simulink model "digital9adder"  (R2024a)
settings: Solver=VariableStepAuto  StartTime=0.0  StopTime=10.0  RelTol=1e-3
settings Model: Creator=tusha  LastModifiedBy=tusha

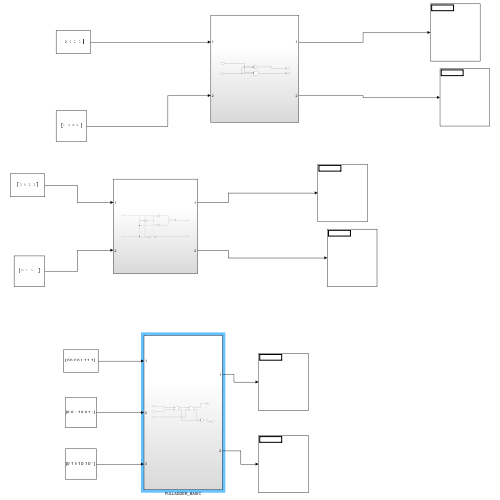
[thumbnail: Simulink's stored preview of the top-level diagram]
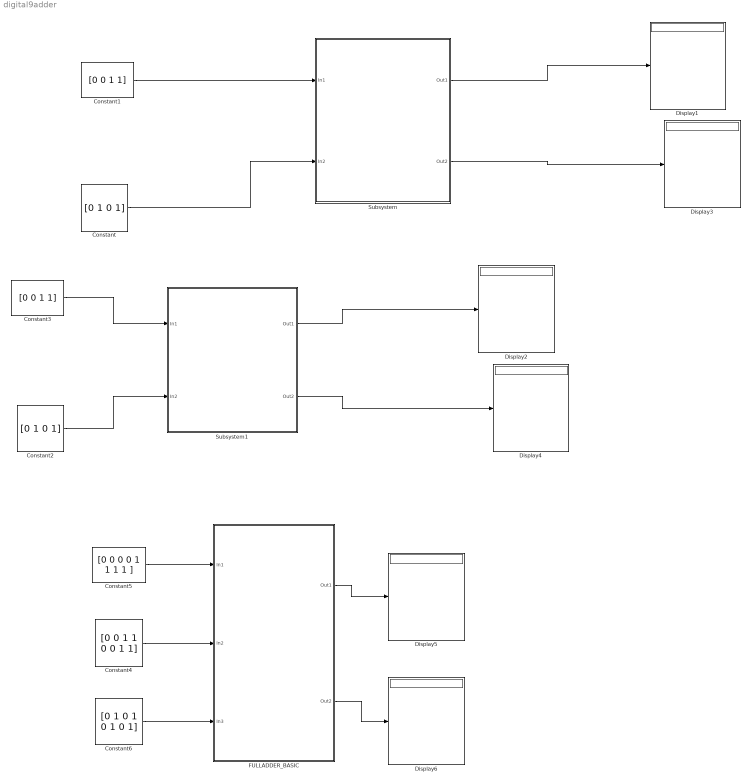
== system digital9adder ==
  Constant : Constant  Value=[0 1 0 1]
  Constant1 : Constant  Value=[0 0 1 1]
  Constant2 : Constant  Value=[0 1 0 1]
  Constant3 : Constant  Value=[0 0 1 1]
  Constant4 : Constant  Value=[0 0 1 1 0 0 1 1]
  Constant5 : Constant  Value=[0 0 0 0 1 1 1 1 ]
  Constant6 : Constant  Value=[0 1 0 1 0 1 0 1]
  Display{1..6} (6 alike) : Display
  FULLADDER_BASIC : Subsystem
  Subsystem : Subsystem
  Subsystem1 : Subsystem
  wires:
  Constant1/1 -> Subsystem/1(In1)
  Constant/1 -> Subsystem/2(In2)
  Subsystem/2(Out2) -> Display3/1
  Subsystem/1(Out1) -> Display1/1
  Constant3/1 -> Subsystem1/1(In1)
  Constant2/1 -> Subsystem1/2(In2)
  Subsystem1/1(Out1) -> Display2/1
  Subsystem1/2(Out2) -> Display4/1
  Constant5/1 -> FULLADDER_BASIC/1(In1)
  Constant4/1 -> FULLADDER_BASIC/2(In2)
  Constant6/1 -> FULLADDER_BASIC/3(In3)
  FULLADDER_BASIC/1(Out1) -> Display5/1
  FULLADDER_BASIC/2(Out2) -> Display6/1

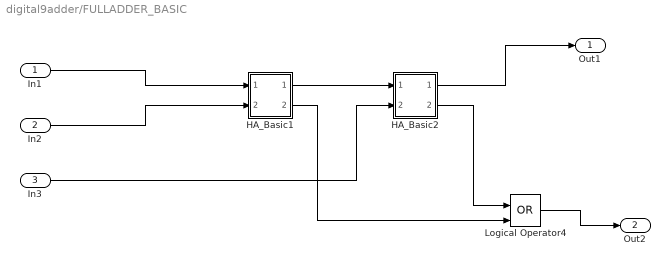
== system digital9adder/FULLADDER_BASIC ==
  In1 : Inport
  In2 : Inport  Port=2
  In3 : Inport  Port=3
  HA_Basic1 : Subsystem
  HA_Basic2 : Subsystem
  Logical Operator4 : Logic  Operator=OR  IconShape=distinctive  AllPortsSameDT=off  OutDataTypeStr=boolean
  Out1 : Outport
  Out2 : Outport  Port=2
  wires:
  HA_Basic1/1(Out1) -> HA_Basic2/1(In1)
  HA_Basic1/2(Out2) -> Logical Operator4/2
  HA_Basic2/2(Out2) -> Logical Operator4/1
  In1/1 -> HA_Basic1/1(In1)
  Logical Operator4/1 -> Out2/1
  In2/1 -> HA_Basic1/2(In2)
  HA_Basic2/1(Out1) -> Out1/1
  In3/1 -> HA_Basic2/2(In2)

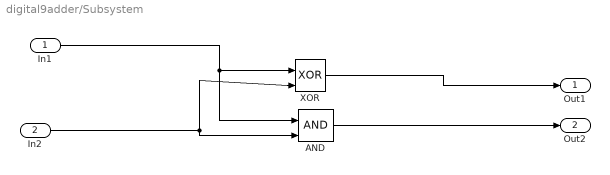
== system digital9adder/Subsystem ==
  In1 : Inport
  In2 : Inport  Port=2
  AND : Logic  IconShape=distinctive  AllPortsSameDT=off  OutDataTypeStr=boolean
  XOR : Logic  Operator=XOR  IconShape=distinctive  AllPortsSameDT=off  OutDataTypeStr=boolean
  Out1 : Outport
  Out2 : Outport  Port=2
  wires:
  In1/1 -> AND/1, XOR/1
  In2/1 -> XOR/2, AND/2
  AND/1 -> Out2/1
  XOR/1 -> Out1/1

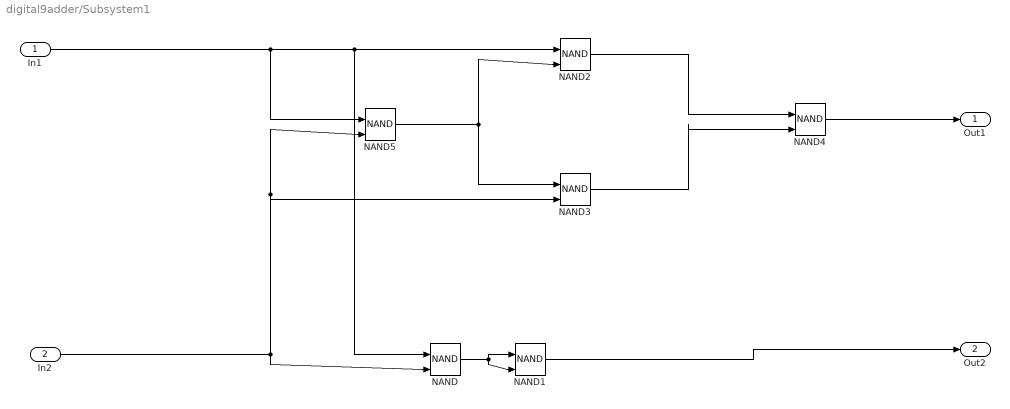
== system digital9adder/Subsystem1 ==
  In1 : Inport
  In2 : Inport  Port=2
  NAND{,1..5} (6 alike) : Logic  Operator=NAND  IconShape=distinctive  AllPortsSameDT=off  OutDataTypeStr=boolean
  Out1 : Outport
  Out2 : Outport  Port=2
  wires:
  In2/1 -> NAND5/2, NAND3/2, NAND/2
  NAND/1 -> NAND1/1, NAND1/2
  NAND1/1 -> Out2/1
  NAND2/1 -> NAND4/1
  NAND3/1 -> NAND4/2
  NAND5/1 -> NAND2/2, NAND3/1
  In1/1 -> NAND/1, NAND2/1, NAND5/1
  NAND4/1 -> Out1/1

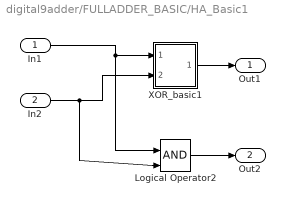
== system digital9adder/FULLADDER_BASIC/HA_Basic1 ==
  In1 : Inport
  In2 : Inport  Port=2
  Logical Operator2 : Logic  IconShape=distinctive  AllPortsSameDT=off  OutDataTypeStr=boolean
  XOR_basic1 : Subsystem
  Out1 : Outport
  Out2 : Outport  Port=2
  wires:
  XOR_basic1/1(Out1) -> Out1/1
  Logical Operator2/1 -> Out2/1
  In1/1 -> Logical Operator2/1, XOR_basic1/1(In1)
  In2/1 -> Logical Operator2/2, XOR_basic1/2(In2)

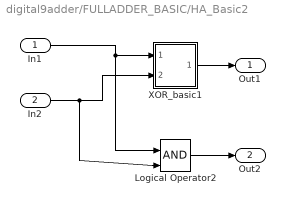
== system digital9adder/FULLADDER_BASIC/HA_Basic2 ==
  In1 : Inport
  In2 : Inport  Port=2
  Logical Operator2 : Logic  IconShape=distinctive  AllPortsSameDT=off  OutDataTypeStr=boolean
  XOR_basic1 : Subsystem
  Out1 : Outport
  Out2 : Outport  Port=2
  wires:
  XOR_basic1/1(Out1) -> Out1/1
  Logical Operator2/1 -> Out2/1
  In1/1 -> Logical Operator2/1, XOR_basic1/1(In1)
  In2/1 -> Logical Operator2/2, XOR_basic1/2(In2)

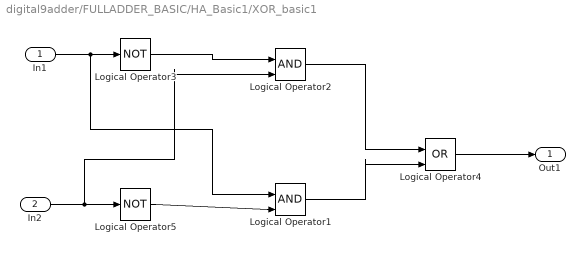
== system digital9adder/FULLADDER_BASIC/HA_Basic1/XOR_basic1 ==
  In1 : Inport
  In2 : Inport  Port=2
  Logical Operator1 : Logic  IconShape=distinctive  AllPortsSameDT=off  OutDataTypeStr=boolean
  Logical Operator2 : Logic  IconShape=distinctive  AllPortsSameDT=off  OutDataTypeStr=boolean
  Logical Operator3 : Logic  Operator=NOT  IconShape=distinctive  AllPortsSameDT=off  OutDataTypeStr=boolean
  Logical Operator4 : Logic  Operator=OR  IconShape=distinctive  AllPortsSameDT=off  OutDataTypeStr=boolean
  Logical Operator5 : Logic  Operator=NOT  IconShape=distinctive  AllPortsSameDT=off  OutDataTypeStr=boolean
  Out1 : Outport
  wires:
  Logical Operator2/1 -> Logical Operator4/1
  Logical Operator3/1 -> Logical Operator2/1
  Logical Operator1/1 -> Logical Operator4/2
  In1/1 -> Logical Operator3/1, Logical Operator1/1
  Logical Operator4/1 -> Out1/1
  Logical Operator5/1 -> Logical Operator1/2
  In2/1 -> Logical Operator2/2, Logical Operator5/1

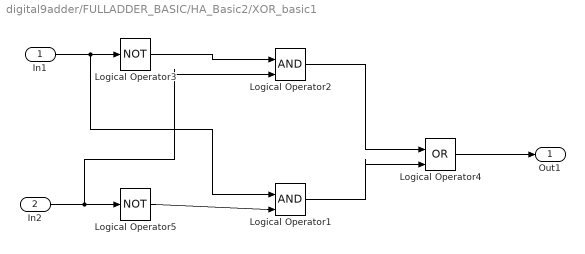
== system digital9adder/FULLADDER_BASIC/HA_Basic2/XOR_basic1 ==
  In1 : Inport
  In2 : Inport  Port=2
  Logical Operator1 : Logic  IconShape=distinctive  AllPortsSameDT=off  OutDataTypeStr=boolean
  Logical Operator2 : Logic  IconShape=distinctive  AllPortsSameDT=off  OutDataTypeStr=boolean
  Logical Operator3 : Logic  Operator=NOT  IconShape=distinctive  AllPortsSameDT=off  OutDataTypeStr=boolean
  Logical Operator4 : Logic  Operator=OR  IconShape=distinctive  AllPortsSameDT=off  OutDataTypeStr=boolean
  Logical Operator5 : Logic  Operator=NOT  IconShape=distinctive  AllPortsSameDT=off  OutDataTypeStr=boolean
  Out1 : Outport
  wires:
  Logical Operator2/1 -> Logical Operator4/1
  Logical Operator3/1 -> Logical Operator2/1
  Logical Operator1/1 -> Logical Operator4/2
  In1/1 -> Logical Operator3/1, Logical Operator1/1
  Logical Operator4/1 -> Out1/1
  Logical Operator5/1 -> Logical Operator1/2
  In2/1 -> Logical Operator2/2, Logical Operator5/1
